simulink model "Sinoatrial"  (R2023b)
settings: Solver=ode23s  StartTime=t(1)  StopTime=t(end)+dt  FixedStep=1  RelTol=1e-2
values from neighbouring files (symbols this model uses):
  params = [ ... (first row only)    [gois09_simulink.m]    (also in ryzhii14_simulink.m; sinoatrial_simulink.m; vdp_simulink.m)
  xInitial = [initial_conditions ... (first row only)    [gois09_simulink.m]    (also in hilaire07martinez_simulink.m = initial_conditions(1:2); jewett99_simulink.m = initial_conditions(1:2); ryzhii14_simulink.m; sinoatrial_simulink.m = initial_conditions)
settings Model: Creator=chukw  LastModifiedBy=chukw
settings DataIOCC: SaveOutput=off  StateSaveName=x  TimeSaveName=t

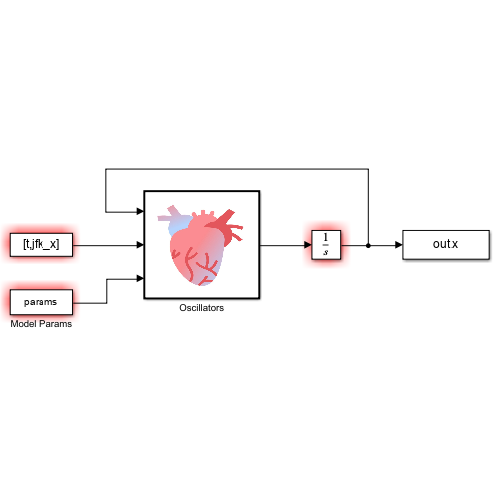
[thumbnail: Simulink's stored preview of the top-level diagram]
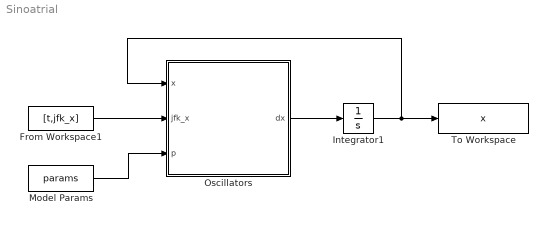
== system Sinoatrial ==
  From Workspace1 : FromWorkspace  VariableName=[t,jfk_x]
  Integrator1 : Integrator  InitialCondition=xInitial
  Model Params : Constant  Value=params
  Oscillators : MATLAB Function  TreatAsAtomicUnit=on
  To Workspace : ToWorkspace  VariableName=x  SampleTime=-1
  wires:
  Oscillators/1(dx) -> Integrator1/1
  Integrator1/1 -> To Workspace/1, Oscillators/1(x)
  Model Params/1 -> Oscillators/3(p)
  From Workspace1/1 -> Oscillators/2(jfk_x)

== matlab function Sinoatrial/Oscillators ==
  data: x input; jfk_x input; dx output; p input
function dx = heart(x, jfk_x, p)
    a1 = p(1);
    u11 = p(2);
    u12 = p(3);
    d1 = p(4);
    e1 = p(5);
    f1 = p(6);
    k_jfk_sa = p(7);

    % Differential equations.
    dx = zeros(2, 1);

    % SA Node.
    dx(1) = x(2);
    dx(2) = (-a1*x(2)*(x(1) - u11)*(x(1) - u12)) -...
        (f1*x(1)*(x(1) + d1)*(x(1) + e1)) + k_jfk_sa*(jfk_x(1) - x(1));
end
